simulink library "hvs_framelib"  (R2016a)
settings: Solver=ode45  StartTime=0.0  StopTime=10.0  RelTol=1e-3
undefined symbols (not defined in the file): aux_power_flag, dcdc_effmap, dcdc_effmap_cooltemp_3rdD, dcdc_effmap_cur_2ndD, dcdc_effmap_vlt_1stD
libraries: Energy_converter_Electrical_to_Mechanical x4, Electrical_converter x2, Energy_converter_Electrical_to_Thermal x1, Electrical_charger x1, Powernet x1, ePTO x1, simulink x1
settings Model: Creator=krishs1  LastModifiedBy=krishs1
settings DataIOCC: LimitDataPoints=on
settings DebuggingCC: AllowSymbolicDim=off

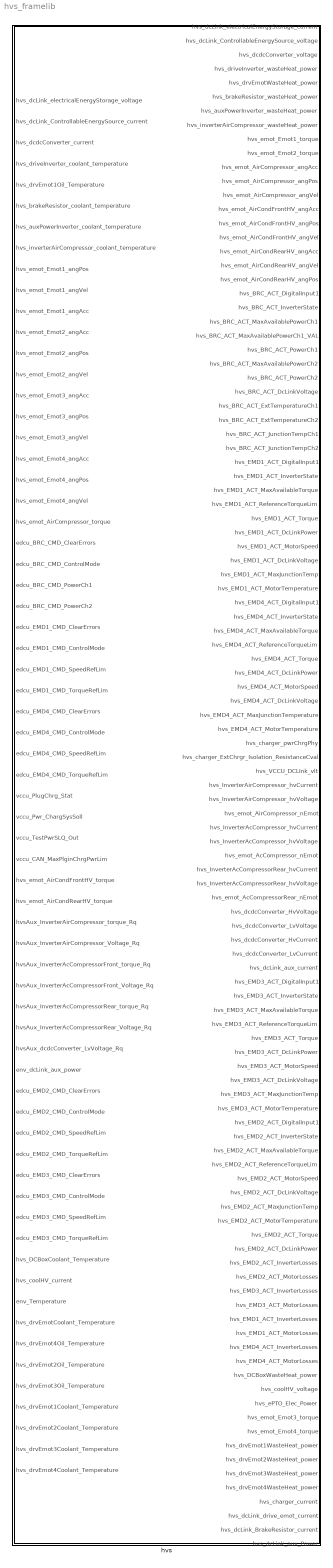
== system hvs_framelib ==
  hvs : Subsystem

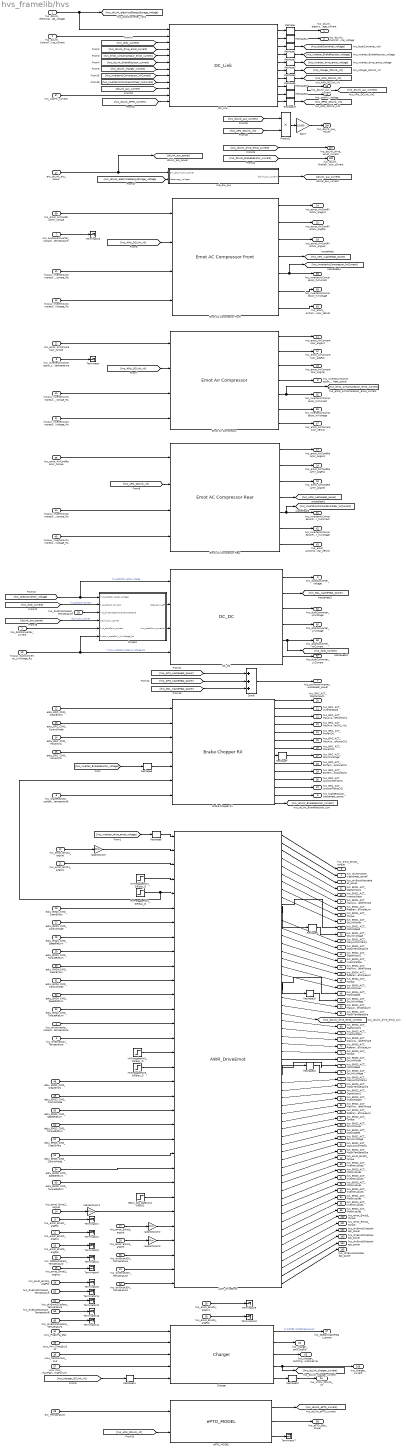
== system hvs_framelib/hvs ==
  hvs_dcLink_electricalEnergyStorage_voltage : Inport
  hvs_dcLink_ControllableEnergySource_current : Inport  Port=2
  hvs_dcdcConverter_current : Inport  Port=3
  hvs_driveInverter_coolant_temperature : Inport  Port=4
  hvs_drvEmot1Oil_Temperature : Inport  Port=5
  hvs_brakeResistor_coolant_temperature : Inport  Port=6
  hvs_auxPowerInverter_coolant_temperature : Inport  Port=7
  hvs_inverterAirCompressor_coolant_temperature : Inport  Port=8
  hvs_emot_Emot1_angPos : Inport  Port=9
  hvs_emot_Emot1_angVel : Inport  Port=10
  hvs_emot_Emot1_angAcc : Inport  Port=11
  hvs_emot_Emot2_angAcc : Inport  Port=12
  hvs_emot_Emot2_angPos : Inport  Port=13
  hvs_emot_Emot2_angVel : Inport  Port=14
  hvs_emot_Emot3_angAcc : Inport  Port=15
  hvs_emot_Emot3_angPos : Inport  Port=16
  hvs_emot_Emot3_angVel : Inport  Port=17
  hvs_emot_Emot4_angAcc : Inport  Port=18
  hvs_emot_Emot4_angPos : Inport  Port=19
  hvs_emot_Emot4_angVel : Inport  Port=20
  hvs_emot_AirCompressor_torque : Inport  Port=21
  edcu_BRC_CMD_ClearErrors : Inport  Port=22
  edcu_BRC_CMD_ControlMode : Inport  Port=23
  edcu_BRC_CMD_PowerCh1 : Inport  Port=24
  edcu_BRC_CMD_PowerCh2 : Inport  Port=25
  edcu_EMD1_CMD_ClearErrors : Inport  Port=26
  edcu_EMD1_CMD_ControlMode : Inport  Port=27
  edcu_EMD1_CMD_SpeedRefLim : Inport  Port=28
  edcu_EMD1_CMD_TorqueRefLim : Inport  Port=29
  edcu_EMD4_CMD_ClearErrors : Inport  Port=30
  edcu_EMD4_CMD_ControlMode : Inport  Port=31
  edcu_EMD4_CMD_SpeedRefLim : Inport  Port=32
  edcu_EMD4_CMD_TorqueRefLim : Inport  Port=33
  vccu_PlugChrg_Stat : Inport  Port=34
  vccu_Pwr_ChargSysSoll : Inport  Port=35
  vccu_TestPwrSLQ_Out : Inport  Port=36
  vccu_CAN_MaxPlginChrgPwrLim : Inport  Port=37
  hvs_emot_AirCondFrontHV_torque : Inport  Port=38
  hvs_emot_AirCondRearHV_torque : Inport  Port=39
  hvsAux_InverterAirCompressor_torque_Rq : Inport  Port=40
  hvsAux_InverterAirCompressor_Voltage_Rq : Inport  Port=41
  hvsAux_InverterAcCompressorFront_torque_Rq : Inport  Port=42
  hvsAux_InverterAcCompressorFront_Voltage_Rq : Inport  Port=43
  hvsAux_InverterAcCompressorRear_torque_Rq : Inport  Port=44
  hvsAux_InverterAcCompressorRear_Voltage_Rq : Inport  Port=45
  hvsAux_dcdcConverter_LvVoltage_Rq : Inport  Port=46
  env_dcLink_aux_power : Inport  Port=47
  edcu_EMD2_CMD_ClearErrors : Inport  Port=48
  edcu_EMD2_CMD_ControlMode : Inport  Port=49
  edcu_EMD2_CMD_SpeedRefLim : Inport  Port=50
  edcu_EMD2_CMD_TorqueRefLim : Inport  Port=51
  edcu_EMD3_CMD_ClearErrors : Inport  Port=52
  edcu_EMD3_CMD_ControlMode : Inport  Port=53
  edcu_EMD3_CMD_SpeedRefLim : Inport  Port=54
  edcu_EMD3_CMD_TorqueRefLim : Inport  Port=55
  hvs_DCBoxCoolant_Temperature : Inport  Port=56
  hvs_coolHV_current : Inport  Port=57
  env_Temperature : Inport  Port=58
  hvs_drvEmotCoolant_Temperature : Inport  Port=59
  hvs_drvEmot4Oil_Temperature : Inport  Port=60
  hvs_drvEmot2Oil_Temperature : Inport  Port=61
  hvs_drvEmot3Oil_Temperature : Inport  Port=62
  hvs_drvEmot1Coolant_Temperature : Inport  Port=63
  hvs_drvEmot2Coolant_Temperature : Inport  Port=64
  hvs_drvEmot3Coolant_Temperature : Inport  Port=65
  hvs_drvEmot4Coolant_Temperature : Inport  Port=66
  AWR_DriveEmot : Energy_converter_Electrical_to_Mechanical/AWR_DriveEmot
  Brake Chopper RX : Energy_converter_Electrical_to_Thermal/Brake Chopper RX
  Charger : Electrical_charger/Charger
  DC_DC : Electrical_converter/DC_DC
  DC_Link : Powernet/DC_Link
  EDCU_Dig_SafetyCutOffDG1 : Step  Time=0.812
  Emot AC Compressor Front : Energy_converter_Electrical_to_Mechanical/Emot AC Compressor Front
  Emot AC Compressor Rear : Energy_converter_Electrical_to_Mechanical/Emot AC Compressor Rear
  Emot Air Compressor : Energy_converter_Electrical_to_Mechanical/Emot Air Compressor
  Gain7 : Gain  Gain=1/1000
  HVFreigabeHW1_SiRelay_D : Step  Time=5.502
  HVFreigabeHW2_SiRelay_D : Step  Time=5.502
  HVFreigabeHW3_SiRelay_D : Step  Time=5.502
  HVFreigabeHW4_SiRelay_D : Step  Time=5.502
  Process : Subsystem
  Product2 : Product  Inputs=**  RndMeth=Zero
  Reshape{,1..17} (18 alike) : Reshape
  Sum8 : Sum  Inputs=+++  SaturateOnIntegerOverflow=on  InputSameDT=on  OutDataTypeStr=Inherit: Same as first input
  Terminator{,1..14} (15 alike) : Terminator
  ePTO_MODEL : ePTO/ePTO_MODEL
  rad/sectorpm{,1..3} (4 alike) : Gain  Gain=30/pi
  sub_env_aux : Subsystem
  hvs_dcLink_electricalEnergyStorage_current : Outport
  hvs_dcLink_ControllableEnergySource_voltage : Outport  Port=2
  hvs_dcdcConverter_voltage : Outport  Port=3
  hvs_driveInverter_wasteHeat_power : Outport  Port=4
  hvs_drvEmotWasteHeat_power : Outport  Port=5
  hvs_brakeResistor_wasteHeat_power : Outport  Port=6
  hvs_auxPowerInverter_wasteHeat_power : Outport  Port=7
  hvs_inverterAirCompressor_wasteHeat_power : Outport  Port=8
  hvs_emot_Emot1_torque : Outport  Port=9
  hvs_emot_Emot2_torque : Outport  Port=10
  hvs_emot_AirCompressor_angAcc : Outport  Port=11
  hvs_emot_AirCompressor_angPos : Outport  Port=12
  hvs_emot_AirCompressor_angVel : Outport  Port=13
  hvs_emot_AirCondFrontHV_angAcc : Outport  Port=14
  hvs_emot_AirCondFrontHV_angPos : Outport  Port=15
  hvs_emot_AirCondFrontHV_angVel : Outport  Port=16
  hvs_emot_AirCondRearHV_angAcc : Outport  Port=17
  hvs_emot_AirCondRearHV_angVel : Outport  Port=18
  hvs_emot_AirCondRearHV_angPos : Outport  Port=19
  hvs_BRC_ACT_DigitalInput1 : Outport  Port=20
  hvs_BRC_ACT_InverterState : Outport  Port=21
  hvs_BRC_ACT_MaxAvailablePowerCh1 : Outport  Port=22
  hvs_BRC_ACT_MaxAvailablePowerCh1_VAL : Outport  Port=23
  hvs_BRC_ACT_PowerCh1 : Outport  Port=24
  hvs_BRC_ACT_MaxAvailablePowerCh2 : Outport  Port=25
  hvs_BRC_ACT_PowerCh2 : Outport  Port=26
  hvs_BRC_ACT_DcLinkVoltage : Outport  Port=27
  hvs_BRC_ACT_ExtTemperatureCh1 : Outport  Port=28
  hvs_BRC_ACT_ExtTemperatureCh2 : Outport  Port=29
  hvs_BRC_ACT_JunctionTempCh1 : Outport  Port=30
  hvs_BRC_ACT_JunctionTempCh2 : Outport  Port=31
  hvs_EMD1_ACT_DigitalInput1 : Outport  Port=32
  hvs_EMD1_ACT_InverterState : Outport  Port=33
  hvs_EMD1_ACT_MaxAvailableTorque : Outport  Port=34
  hvs_EMD1_ACT_ReferenceTorqueLim : Outport  Port=35
  hvs_EMD1_ACT_Torque : Outport  Port=36
  hvs_EMD1_ACT_DcLinkPower : Outport  Port=37
  hvs_EMD1_ACT_MotorSpeed : Outport  Port=38
  hvs_EMD1_ACT_DcLinkVoltage : Outport  Port=39
  hvs_EMD1_ACT_MaxJunctionTemp : Outport  Port=40
  hvs_EMD1_ACT_MotorTemperature : Outport  Port=41
  hvs_EMD4_ACT_DigitalInput1 : Outport  Port=42
  hvs_EMD4_ACT_InverterState : Outport  Port=43
  hvs_EMD4_ACT_MaxAvailableTorque : Outport  Port=44
  hvs_EMD4_ACT_ReferenceTorqueLim : Outport  Port=45
  hvs_EMD4_ACT_Torque : Outport  Port=46
  hvs_EMD4_ACT_DcLinkPower : Outport  Port=47
  hvs_EMD4_ACT_MotorSpeed : Outport  Port=48
  hvs_EMD4_ACT_DcLinkVoltage : Outport  Port=49
  hvs_EMD4_ACT_MaxJunctionTemperature : Outport  Port=50
  hvs_EMD4_ACT_MotorTemperature : Outport  Port=51
  hvs_charger_pwrChrgPhy : Outport  Port=52
  hvs_charger_ExtChrgr_Isolation_ResistanceCval : Outport  Port=53
  hvs_VCCU_DCLInk_vlt : Outport  Port=54
  hvs_InverterAirCompressor_hvCurrent : Outport  Port=55
  hvs_InverterAirCompressor_hvVoltage : Outport  Port=56
  hvs_emot_AirCompressor_nEmot : Outport  Port=57
  hvs_InverterAcCompressor_hvCurrent : Outport  Port=58
  hvs_InverterAcCompressor_hvVoltage : Outport  Port=59
  hvs_emot_AcCompressor_nEmot : Outport  Port=60
  hvs_InverterAcCompressorRear_hvCurrent : Outport  Port=61
  hvs_InverterAcCompressorRear_hvVoltage : Outport  Port=62
  hvs_emot_AcCompressorRear_nEmot : Outport  Port=63
  hvs_dcdcConverter_HvVoltage : Outport  Port=64
  hvs_dcdcConverter_LvVoltage : Outport  Port=65
  hvs_dcdcConverter_HvCurrent : Outport  Port=66
  hvs_dcdcConverter_LvCurrent : Outport  Port=67
  hvs_dcLink_aux_current : Outport  Port=68
  hvs_EMD3_ACT_DigitalInput1 : Outport  Port=69
  hvs_EMD3_ACT_InverterState : Outport  Port=70
  hvs_EMD3_ACT_MaxAvailableTorque : Outport  Port=71
  hvs_EMD3_ACT_ReferenceTorqueLim : Outport  Port=72
  hvs_EMD3_ACT_Torque : Outport  Port=73
  hvs_EMD3_ACT_DcLinkPower : Outport  Port=74
  hvs_EMD3_ACT_MotorSpeed : Outport  Port=75
  hvs_EMD3_ACT_DcLinkVoltage : Outport  Port=76
  hvs_EMD3_ACT_MaxJunctionTemp : Outport  Port=77
  hvs_EMD3_ACT_MotorTemperature : Outport  Port=78
  hvs_EMD2_ACT_DigitalInput1 : Outport  Port=79
  hvs_EMD2_ACT_InverterState : Outport  Port=80
  hvs_EMD2_ACT_MaxAvailableTorque : Outport  Port=81
  hvs_EMD2_ACT_ReferenceTorqueLim : Outport  Port=82
  hvs_EMD2_ACT_MotorSpeed : Outport  Port=83
  hvs_EMD2_ACT_DcLinkVoltage : Outport  Port=84
  hvs_EMD2_ACT_MaxJunctionTemp : Outport  Port=85
  hvs_EMD2_ACT_MotorTemperature : Outport  Port=86
  hvs_EMD2_ACT_Torque : Outport  Port=87
  hvs_EMD2_ACT_DcLinkPower : Outport  Port=88
  hvs_EMD2_ACT_InverterLosses : Outport  Port=89
  hvs_EMD2_ACT_MotorLosses : Outport  Port=90
  hvs_EMD3_ACT_InverterLosses : Outport  Port=91
  hvs_EMD3_ACT_MotorLosses : Outport  Port=92
  hvs_EMD1_ACT_InverterLosses : Outport  Port=93
  hvs_EMD1_ACT_MotorLosses : Outport  Port=94
  hvs_EMD4_ACT_InverterLosses : Outport  Port=95
  hvs_EMD4_ACT_MotorLosses : Outport  Port=96
  hvs_DCBoxWasteHeat_power : Outport  Port=97
  hvs_coolHV_voltage : Outport  Port=98
  hvs_ePTO_Elec_Power : Outport  Port=99
  hvs_emot_Emot3_torque : Outport  Port=100
  hvs_emot_Emot4_torque : Outport  Port=101
  hvs_drvEmot1WasteHeat_power : Outport  Port=102
  hvs_drvEmot2WasteHeat_power : Outport  Port=103
  hvs_drvEmot3WasteHeat_power : Outport  Port=104
  hvs_drvEmot4WasteHeat_power : Outport  Port=105
  hvs_charger_current : Outport  Port=106
  hvs_dcLink_drive_emot_current : Outport  Port=107
  hvs_dcLink_BrakeResistor_current : Outport  Port=108
  hvs_dcLink_aux_Power : Outport  Port=109
  wires:
  Gain7/1 -> hvs_dcLink_aux_Power/1
  Product2/1 -> Gain7/1
  [hvs_APIs_DCLink_vlt] -> Product2/2
  [hvs_dcLink_aux_current] -> Product2/1
  [hvs_dcLink_BrakeResistor_current] -> hvs_dcLink_BrakeResistor_current/1
  [hvs_dcLink_drive_emot_current] -> hvs_dcLink_drive_emot_current/1
  AWR_DriveEmot/59 -> hvs_drvEmot4WasteHeat_power/1
  AWR_DriveEmot/58 -> hvs_drvEmot3WasteHeat_power/1
  AWR_DriveEmot/57 -> hvs_drvEmot2WasteHeat_power/1
  AWR_DriveEmot/56 -> hvs_drvEmot1WasteHeat_power/1
  AWR_DriveEmot/55 -> hvs_emot_Emot4_torque/1
  AWR_DriveEmot/54 -> hvs_emot_Emot3_torque/1
  AWR_DriveEmot/24 -> [hvs_dcLink_drive_emot_current]
  hvs_drvEmot4Coolant_Temperature/1 -> Terminator14/1
  hvs_drvEmot3Coolant_Temperature/1 -> Terminator13/1
  hvs_drvEmot2Coolant_Temperature/1 -> Terminator12/1
  hvs_drvEmot1Coolant_Temperature/1 -> Terminator11/1
  hvs_drvEmot3Oil_Temperature/1 -> AWR_DriveEmot/32
  hvs_drvEmot2Oil_Temperature/1 -> AWR_DriveEmot/31
  hvs_drvEmot4Oil_Temperature/1 -> AWR_DriveEmot/30
  AWR_DriveEmot/4 -> hvs_EMD1_ACT_DigitalInput1/1
  rad/sectorpm3/1 -> AWR_DriveEmot/29
  rad/sectorpm2/1 -> AWR_DriveEmot/28
  hvs_emot_Emot3_angVel/1 -> rad/sectorpm2/1
  hvs_emot_Emot4_angVel/1 -> rad/sectorpm3/1
  hvs_emot_Emot4_angPos/1 -> Terminator10/1
  hvs_emot_Emot4_angAcc/1 -> Terminator9/1
  hvs_emot_Emot3_angPos/1 -> Terminator8/1
  hvs_emot_Emot3_angAcc/1 -> Terminator6/1
  Process/2(hvs_dcdcConv_current1) -> DC_DC/3
  Process/1(dcdc_conv_eff) -> DC_DC/2
  hvs_dcdcConverter_current/1 -> Process/5(hvs_dcdcConv_current)
  [dcLink_aux_power] -> Process/4(dcLink_aux_power)  "dcLink_aux_power"
  hvs_drvEmotCoolant_Temperature/1 -> Process/3(hvs_drvEmotCoolant_Temperature)
  [hvs_dcdc_current] -> Process/2(hvs_dcdc_HvCurrent)  "hvs_dcdc_HvCurrent"
  [hvs_dcLink_ePTO_current] -> DC_Link/12
  [hvs_APIs_DCLink_vlt] -> ePTO_MODEL/2
  ePTO_MODEL/3 -> Terminator7/1
  ePTO_MODEL/2 -> hvs_ePTO_Elec_Power/1
  ePTO_MODEL/1 -> [hvs_dcLink_ePTO_current]
  DC_Link/10 -> Reshape17/1
  Reshape17/1 -> [hvs_ePTO_DCLink_vlt]
  env_Temperature/1 -> ePTO_MODEL/1
  hvs_DCBoxCoolant_Temperature/1 -> Terminator4/1
  Charger/1 -> hvs_DCBoxWasteHeat_power/1  "hvs_DCBoxWasteHeat_power"
  hvsAux_dcdcConverter_LvVoltage_Rq/1 -> DC_DC/4, Process/6(hvsAux_dcdcConv_LvVoltage_Rq)  "hvsAux_dcdcConverter_LvVoltage_Rq"
  DC_Link/8 -> Reshape15/1
  [hvs_dcLink_electricalEnergyStorage_voltage] -> sub_env_aux/2(Nebenagg_voltage)
  sub_env_aux/1(dcLink_aux_current) -> [dcLink_aux_current]
  env_dcLink_aux_power/1 -> sub_env_aux/1(env_dcLink_aux_power), [dcLink_aux_power]
  [dcLink_aux_current] -> DC_Link/10
  Reshape12/1 -> hvs_VCCU_DCLInk_vlt/1
  Reshape11/1 -> Charger/5
  Reshape10/1 -> hvs_EMD4_ACT_DcLinkVoltage/1
  Reshape8/1 -> AWR_DriveEmot/1
  Reshape7/1 -> hvs_BRC_ACT_DcLinkVoltage/1
  Reshape6/1 -> Brake Chopper RX/5
  Reshape5/1 -> [hvs_APIs_DCLink_vlt]
  Reshape4/1 -> [hvs_charger_DCLink_vlt]
  Reshape3/1 -> [hvs_inverter_drive_emot_voltage]
  Reshape2/1 -> [hvs_inverter_BrakeResistor_voltage]
  Reshape1/1 -> [hvs_dcdcConverter_voltage]
  Reshape/1 -> hvs_dcLink_electricalEnergyStorage_current/1
  rad/sectorpm/1 -> AWR_DriveEmot/2
  [hvs_dcdc_current] -> DC_Link/3
  [hvs_DCL_wasteHeat_power] -> Sum8/3
  [hvs_API3_wasteHeat_power] -> Sum8/2
  [hvs_API1_wasteHeat_power] -> Sum8/1
  Sum8/1 -> hvs_auxPowerInverter_wasteHeat_power/1
  DC_DC/6 -> hvs_dcdcConverter_LvCurrent/1
  DC_DC/5 -> hvs_dcdcConverter_HvCurrent/1, [hvs_dcdc_current]
  DC_DC/4 -> hvs_dcdcConverter_LvVoltage/1
  DC_DC/3 -> hvs_dcdcConverter_HvVoltage/1
  DC_Link/3 -> Reshape1/1
  DC_DC/1 -> hvs_dcdcConverter_voltage/1
  DC_DC/2 -> [hvs_DCL_wasteHeat_power]
  [hvs_dcdcConverter_voltage] -> Process/1(hvs_dcdcConverter_voltage), DC_DC/1  "hvs_dcdcConverter_voltage"
  Emot AC Compressor Rear/4 -> [hvs_API3_wasteHeat_power]
  Emot AC Compressor Rear/5 -> [hvs_InverterAcCompressorRear_hvCurrent], hvs_InverterAcCompressorRear_hvCurrent/1
  Emot AC Compressor Rear/6 -> hvs_InverterAcCompressorRear_hvVoltage/1
  Emot AC Compressor Rear/7 -> hvs_emot_AcCompressorRear_nEmot/1
  Emot AC Compressor Rear/2 -> hvs_emot_AirCondRearHV_angPos/1
  Emot AC Compressor Rear/3 -> hvs_emot_AirCondRearHV_angVel/1
  Emot AC Compressor Rear/1 -> hvs_emot_AirCondRearHV_angAcc/1
  hvsAux_InverterAcCompressorRear_Voltage_Rq/1 -> Emot AC Compressor Rear/4
  hvsAux_InverterAcCompressorRear_torque_Rq/1 -> Emot AC Compressor Rear/3
  [hvs_APIs_DCLink_vlt] -> Emot AC Compressor Rear/2
  hvs_emot_AirCondRearHV_torque/1 -> Emot AC Compressor Rear/1
  Emot AC Compressor Front/4 -> [hvs_API1_wasteHeat_power]
  Emot AC Compressor Front/6 -> hvs_InverterAcCompressor_hvVoltage/1
  Emot AC Compressor Front/7 -> hvs_emot_AcCompressor_nEmot/1
  Emot AC Compressor Front/3 -> hvs_emot_AirCondFrontHV_angVel/1
  Emot AC Compressor Front/2 -> hvs_emot_AirCondFrontHV_angPos/1
  Emot AC Compressor Front/1 -> hvs_emot_AirCondFrontHV_angAcc/1
  hvsAux_InverterAcCompressorFront_Voltage_Rq/1 -> Emot AC Compressor Front/4
  hvsAux_InverterAcCompressorFront_torque_Rq/1 -> Emot AC Compressor Front/3
  hvs_emot_AirCondFrontHV_torque/1 -> Emot AC Compressor Front/1
  [hvs_APIs_DCLink_vlt] -> Emot AC Compressor Front/2
  hvs_auxPowerInverter_coolant_temperature/1 -> Terminator5/1
  hvs_inverterAirCompressor_coolant_temperature/1 -> Terminator/1
  hvsAux_InverterAirCompressor_Voltage_Rq/1 -> Emot Air Compressor/4
  hvsAux_InverterAirCompressor_torque_Rq/1 -> Emot Air Compressor/3
  [hvs_APIs_DCLink_vlt] -> Emot Air Compressor/2
  DC_Link/7 -> Reshape5/1
  Emot Air Compressor/6 -> hvs_InverterAirCompressor_hvVoltage/1
  Emot Air Compressor/7 -> hvs_emot_AirCompressor_nEmot/1
  Emot Air Compressor/5 -> [hvs_emot_AirCompressor_emot_current], hvs_InverterAirCompressor_hvCurrent/1
  Emot Air Compressor/4 -> hvs_inverterAirCompressor_wasteHeat_power/1
  Emot Air Compressor/3 -> hvs_emot_AirCompressor_angVel/1
  Emot Air Compressor/2 -> hvs_emot_AirCompressor_angPos/1
  Emot Air Compressor/1 -> hvs_emot_AirCompressor_angAcc/1
  hvs_emot_AirCompressor_torque/1 -> Emot Air Compressor/1
  DC_Link/1 -> Reshape/1
  DC_Link/2 -> Reshape14/1
  hvs_dcLink_electricalEnergyStorage_voltage/1 -> [hvs_dcLink_electricalEnergyStorage_voltage], DC_Link/1
  hvs_dcLink_ControllableEnergySource_current/1 -> DC_Link/2
  edcu_BRC_CMD_ClearErrors/1 -> Brake Chopper RX/1
  edcu_BRC_CMD_ControlMode/1 -> Brake Chopper RX/2
  edcu_BRC_CMD_PowerCh1/1 -> Brake Chopper RX/3
  edcu_BRC_CMD_PowerCh2/1 -> Brake Chopper RX/4
  DC_Link/4 -> Reshape2/1
  Brake Chopper RX/1 -> hvs_BRC_ACT_DigitalInput1/1
  Brake Chopper RX/2 -> hvs_BRC_ACT_InverterState/1
  Brake Chopper RX/3 -> hvs_BRC_ACT_MaxAvailablePowerCh1/1
  Brake Chopper RX/4 -> hvs_BRC_ACT_MaxAvailablePowerCh1_VAL/1
  Brake Chopper RX/5 -> hvs_BRC_ACT_PowerCh1/1
  Brake Chopper RX/6 -> hvs_BRC_ACT_MaxAvailablePowerCh2/1
  Brake Chopper RX/7 -> hvs_BRC_ACT_PowerCh2/1
  Brake Chopper RX/8 -> Reshape7/1
  Brake Chopper RX/9 -> hvs_BRC_ACT_ExtTemperatureCh1/1
  Brake Chopper RX/10 -> hvs_BRC_ACT_ExtTemperatureCh2/1
  Brake Chopper RX/11 -> hvs_BRC_ACT_JunctionTempCh1/1
  Brake Chopper RX/12 -> hvs_BRC_ACT_JunctionTempCh2/1
  [hvs_inverter_BrakeResistor_voltage] -> Reshape6/1
  hvs_emot_Emot1_angVel/1 -> rad/sectorpm/1
  hvs_emot_Emot1_angAcc/1 -> AWR_DriveEmot/3
  DC_Link/5 -> Reshape3/1
  [hvs_inverter_drive_emot_voltage] -> Reshape8/1
  [hvs_dcLink_drive_emot_current] -> DC_Link/4
  [hvs_emot_AirCompressor_emot_current] -> DC_Link/5
  Brake Chopper RX/13 -> hvs_brakeResistor_wasteHeat_power/1
  hvs_brakeResistor_coolant_temperature/1 -> Brake Chopper RX/7
  HVFreigabeHW4_SiRelay_D/1 -> AWR_DriveEmot/5, Brake Chopper RX/6
  Brake Chopper RX/14 -> [hvs_dcLink_BrakeResistor_current]
  [hvs_dcLink_BrakeResistor_current] -> DC_Link/6
  HVFreigabeHW1_SiRelay_D/1 -> AWR_DriveEmot/4
  hvs_drvEmot1Oil_Temperature/1 -> AWR_DriveEmot/15
  hvs_driveInverter_coolant_temperature/1 -> AWR_DriveEmot/14
  hvs_emot_Emot1_angPos/1 -> Terminator1/1
  hvs_emot_Emot2_angAcc/1 -> Terminator2/1
  hvs_emot_Emot2_angPos/1 -> Terminator3/1
  hvs_emot_Emot2_angVel/1 -> rad/sectorpm1/1
  AWR_DriveEmot/45 -> hvs_emot_Emot2_torque/1
  AWR_DriveEmot/11 -> Reshape9/1
  AWR_DriveEmot/12 -> hvs_EMD1_ACT_MaxJunctionTemp/1
  AWR_DriveEmot/13 -> hvs_EMD1_ACT_MotorTemperature/1
  AWR_DriveEmot/14 -> hvs_EMD4_ACT_DigitalInput1/1
  AWR_DriveEmot/15 -> hvs_EMD4_ACT_InverterState/1
  AWR_DriveEmot/16 -> hvs_EMD4_ACT_MaxAvailableTorque/1
  AWR_DriveEmot/17 -> hvs_EMD4_ACT_ReferenceTorqueLim/1
  AWR_DriveEmot/18 -> hvs_EMD4_ACT_Torque/1
  AWR_DriveEmot/19 -> hvs_EMD4_ACT_DcLinkPower/1
  AWR_DriveEmot/20 -> hvs_EMD4_ACT_MotorSpeed/1
  AWR_DriveEmot/21 -> Reshape10/1
  AWR_DriveEmot/22 -> hvs_EMD4_ACT_MaxJunctionTemperature/1
  AWR_DriveEmot/23 -> hvs_EMD4_ACT_MotorTemperature/1
  edcu_EMD1_CMD_ClearErrors/1 -> AWR_DriveEmot/6
  edcu_EMD1_CMD_ControlMode/1 -> AWR_DriveEmot/7
  edcu_EMD1_CMD_SpeedRefLim/1 -> AWR_DriveEmot/8
  edcu_EMD1_CMD_TorqueRefLim/1 -> AWR_DriveEmot/9
  edcu_EMD4_CMD_ClearErrors/1 -> AWR_DriveEmot/10
  edcu_EMD4_CMD_ControlMode/1 -> AWR_DriveEmot/11
  edcu_EMD4_CMD_SpeedRefLim/1 -> AWR_DriveEmot/12
  edcu_EMD4_CMD_TorqueRefLim/1 -> AWR_DriveEmot/13
  vccu_CAN_MaxPlginChrgPwrLim/1 -> Charger/4
  [hvs_charger_DCLink_vlt] -> Reshape11/1
  vccu_TestPwrSLQ_Out/1 -> Charger/3
  vccu_Pwr_ChargSysSoll/1 -> Charger/2
  vccu_PlugChrg_Stat/1 -> Charger/1
  Charger/2 -> hvs_charger_pwrChrgPhy/1
  Charger/3 -> hvs_charger_ExtChrgr_Isolation_ResistanceCval/1
  Charger/4 -> [hvs_dcLink_charger_current], hvs_charger_current/1
  [hvs_dcLink_charger_current] -> DC_Link/7
  DC_Link/6 -> Reshape4/1
  Charger/5 -> Reshape12/1
  Emot AC Compressor Front/5 -> [hvs_InverterAcCompressor_hvCurrent], hvs_InverterAcCompressor_hvCurrent/1
  [hvs_InverterAcCompressor_hvCurrent] -> DC_Link/8
  [hvs_InverterAcCompressorRear_hvCurrent] -> DC_Link/9
  AWR_DriveEmot/1 -> hvs_emot_Emot1_torque/1
  AWR_DriveEmot/2 -> hvs_driveInverter_wasteHeat_power/1
  AWR_DriveEmot/3 -> hvs_drvEmotWasteHeat_power/1
  AWR_DriveEmot/5 -> hvs_EMD1_ACT_InverterState/1
  AWR_DriveEmot/6 -> hvs_EMD1_ACT_MaxAvailableTorque/1
  AWR_DriveEmot/7 -> hvs_EMD1_ACT_ReferenceTorqueLim/1
  AWR_DriveEmot/8 -> hvs_EMD1_ACT_Torque/1
  AWR_DriveEmot/9 -> hvs_EMD1_ACT_DcLinkPower/1
  Reshape9/1 -> hvs_EMD1_ACT_DcLinkVoltage/1
  AWR_DriveEmot/10 -> hvs_EMD1_ACT_MotorSpeed/1
  AWR_DriveEmot/32 -> Reshape13/1
  AWR_DriveEmot/33 -> hvs_EMD3_ACT_MaxJunctionTemp/1
  AWR_DriveEmot/34 -> hvs_EMD3_ACT_MotorTemperature/1
  AWR_DriveEmot/35 -> hvs_EMD2_ACT_DigitalInput1/1
  AWR_DriveEmot/26 -> hvs_EMD3_ACT_InverterState/1
  AWR_DriveEmot/27 -> hvs_EMD3_ACT_MaxAvailableTorque/1
  AWR_DriveEmot/28 -> hvs_EMD3_ACT_ReferenceTorqueLim/1
  AWR_DriveEmot/29 -> hvs_EMD3_ACT_Torque/1
  AWR_DriveEmot/30 -> hvs_EMD3_ACT_DcLinkPower/1
  Reshape13/1 -> hvs_EMD3_ACT_DcLinkVoltage/1
  AWR_DriveEmot/31 -> hvs_EMD3_ACT_MotorSpeed/1
  AWR_DriveEmot/25 -> hvs_EMD3_ACT_DigitalInput1/1
  AWR_DriveEmot/36 -> hvs_EMD2_ACT_InverterState/1
  AWR_DriveEmot/37 -> hvs_EMD2_ACT_MaxAvailableTorque/1
  AWR_DriveEmot/38 -> hvs_EMD2_ACT_ReferenceTorqueLim/1
  AWR_DriveEmot/41 -> hvs_EMD2_ACT_MotorSpeed/1
  AWR_DriveEmot/42 -> hvs_EMD2_ACT_DcLinkVoltage/1
  AWR_DriveEmot/43 -> hvs_EMD2_ACT_MaxJunctionTemp/1
  AWR_DriveEmot/44 -> hvs_EMD2_ACT_MotorTemperature/1
  AWR_DriveEmot/39 -> hvs_EMD2_ACT_Torque/1
  AWR_DriveEmot/40 -> hvs_EMD2_ACT_DcLinkPower/1
  EDCU_Dig_SafetyCutOffDG1/1 -> AWR_DriveEmot/26
  HVFreigabeHW2_SiRelay_D/1 -> AWR_DriveEmot/16
  HVFreigabeHW3_SiRelay_D/1 -> AWR_DriveEmot/17
  rad/sectorpm1/1 -> AWR_DriveEmot/27
  edcu_EMD3_CMD_ControlMode/1 -> AWR_DriveEmot/23
  edcu_EMD2_CMD_ClearErrors/1 -> AWR_DriveEmot/18
  edcu_EMD2_CMD_ControlMode/1 -> AWR_DriveEmot/19
  edcu_EMD2_CMD_SpeedRefLim/1 -> AWR_DriveEmot/20
  edcu_EMD2_CMD_TorqueRefLim/1 -> AWR_DriveEmot/21
  edcu_EMD3_CMD_ClearErrors/1 -> AWR_DriveEmot/22
  edcu_EMD3_CMD_SpeedRefLim/1 -> AWR_DriveEmot/24
  edcu_EMD3_CMD_TorqueRefLim/1 -> AWR_DriveEmot/25
  AWR_DriveEmot/46 -> hvs_EMD2_ACT_InverterLosses/1
  AWR_DriveEmot/47 -> hvs_EMD2_ACT_MotorLosses/1
  AWR_DriveEmot/48 -> hvs_EMD3_ACT_InverterLosses/1
  AWR_DriveEmot/49 -> hvs_EMD3_ACT_MotorLosses/1
  AWR_DriveEmot/50 -> hvs_EMD1_ACT_InverterLosses/1
  AWR_DriveEmot/51 -> hvs_EMD1_ACT_MotorLosses/1
  AWR_DriveEmot/52 -> hvs_EMD4_ACT_InverterLosses/1
  AWR_DriveEmot/53 -> hvs_EMD4_ACT_MotorLosses/1
  Reshape14/1 -> hvs_dcLink_ControllableEnergySource_voltage/1
  Reshape15/1 -> hvs_dcLink_aux_current/1, [hvs_dcLink_aux_current]
  DC_Link/9 -> Reshape16/1
  Reshape16/1 -> hvs_coolHV_voltage/1
  hvs_coolHV_current/1 -> DC_Link/11

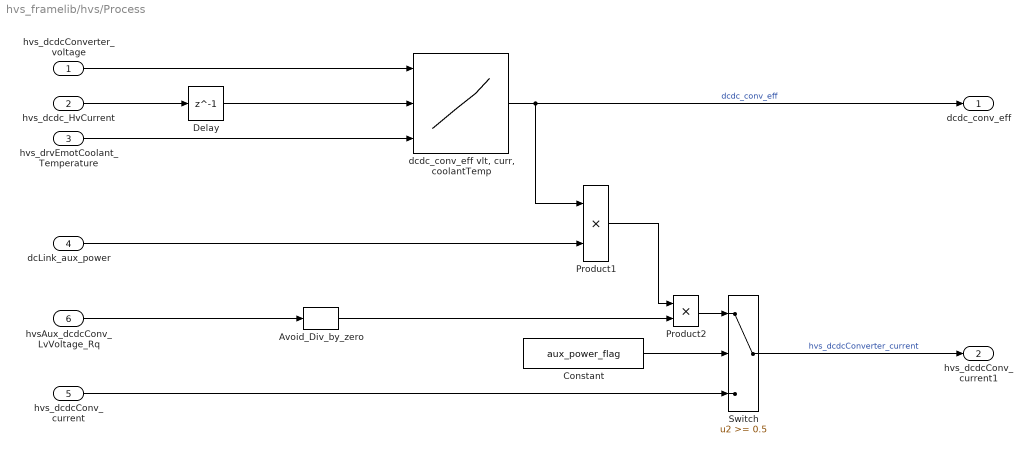
== system hvs_framelib/hvs/Process ==
  hvs_dcdcConverter_voltage : Inport
  hvs_dcdc_HvCurrent : Inport  Port=2
  hvs_drvEmotCoolant_Temperature : Inport  Port=3
  dcLink_aux_power : Inport  Port=4
  hvs_dcdcConv_current : Inport  Port=5
  hvsAux_dcdcConv_LvVoltage_Rq : Inport  Port=6
  Avoid_Div_by_zero : Electrical_converter/DC_DC/Avoid_Div_by_zero
  Constant : Constant  Value=aux_power_flag
  Delay : Delay  DelayLength=1  InitialCondition=0
  Product1 : Product  Inputs=**  RndMeth=Zero
  Product2 : Product  Inputs=**  RndMeth=Zero
  Switch : Switch  Threshold=0.5
  "dcdc_conv_eff vlt, curr, coolantTemp" : Lookup_n-D  NumberOfTableDimensions=3  BreakpointsForDimension1=dcdc_effmap_vlt_1stD  BreakpointsForDimension2=dcdc_effmap_cur_2ndD  BreakpointsForDimension3=dcdc_effmap_cooltemp_3rdD  Table=dcdc_effmap  ExtrapMethod=Clip  RndMeth=Simplest  InputSameDT=on
  dcdc_conv_eff : Outport
  hvs_dcdcConv_current1 : Outport  Port=2
  wires:
  Delay/1 -> "dcdc_conv_eff vlt, curr, coolantTemp"/2
  hvs_dcdc_HvCurrent/1 -> Delay/1
  "dcdc_conv_eff vlt, curr, coolantTemp"/1 -> dcdc_conv_eff/1, Product1/1  "dcdc_conv_eff"
  Product2/1 -> Switch/1
  Product1/1 -> Product2/1
  hvs_dcdcConv_current/1 -> Switch/3
  Switch/1 -> hvs_dcdcConv_current1/1  "hvs_dcdcConverter_current"
  dcLink_aux_power/1 -> Product1/2
  Avoid_Div_by_zero/1 -> Product2/2
  Constant/1 -> Switch/2
  hvsAux_dcdcConv_LvVoltage_Rq/1 -> Avoid_Div_by_zero/1
  hvs_dcdcConverter_voltage/1 -> "dcdc_conv_eff vlt, curr, coolantTemp"/1
  hvs_drvEmotCoolant_Temperature/1 -> "dcdc_conv_eff vlt, curr, coolantTemp"/3

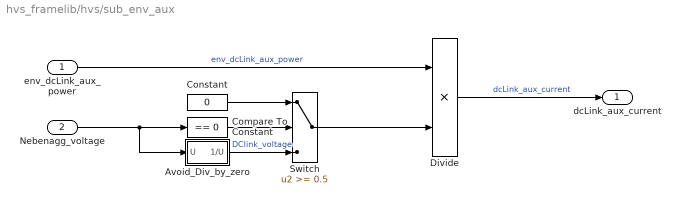
== system hvs_framelib/hvs/sub_env_aux ==
  env_dcLink_aux_power : Inport
  Nebenagg_voltage : Inport  Port=2
  Avoid_Div_by_zero : Subsystem
  Compare To Constant : simulink/Logic and Bit Operations/Compare To Constant  relop===  const=0  OutDataTypeStr=boolean
  Constant : Constant  Value=0
  Divide : Product
  Switch : Switch  Threshold=0.5
  dcLink_aux_current : Outport
  wires:
  Divide/1 -> dcLink_aux_current/1  "dcLink_aux_current"
  Nebenagg_voltage/1 -> Avoid_Div_by_zero/1(U), Compare To Constant/1
  Avoid_Div_by_zero/1(1/U) -> Switch/3  "DClink_voltage"
  env_dcLink_aux_power/1 -> Divide/1  "env_dcLink_aux_power"
  Compare To Constant/1 -> Switch/2
  Constant/1 -> Switch/1
  Switch/1 -> Divide/2

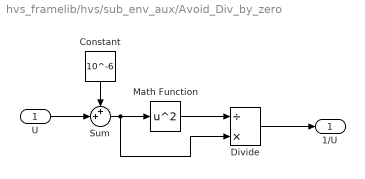
== system hvs_framelib/hvs/sub_env_aux/Avoid_Div_by_zero ==
  U : Inport
  Constant : Constant  Value=10^-6
  Divide : Product  Inputs=/*
  Math Function : Math  Operator=square  SaturateOnIntegerOverflow=on
  Sum : Sum  Inputs=++|
  1/U : Outport
  wires:
  U/1 -> Sum/2
  Constant/1 -> Sum/1
  Sum/1 -> Math Function/1, Divide/2
  Math Function/1 -> Divide/1
  Divide/1 -> 1/U/1
